simulink model "open_loop"  (R2021b)
settings: Solver=VariableStepAuto  StartTime=0.0  StopTime=2  RelTol=1e-3
undefined symbols (not defined in the file or in its folder): A, B, C, D
settings Model: Creator=Dawson  LastModifiedBy=Dawson

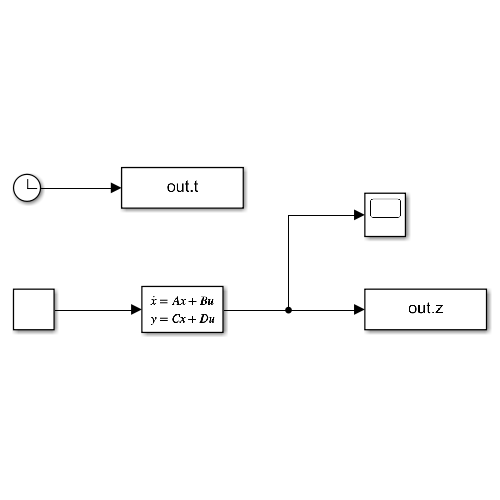
[thumbnail: Simulink's stored preview of the top-level diagram]
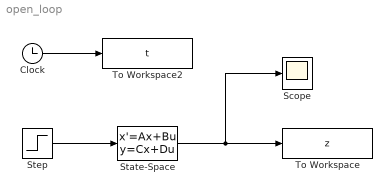
== system open_loop ==
  Clock : Clock
  Scope : Scope
  State-Space : StateSpace  A=A  B=B  C=C  D=D  InitialCondition=0
  Step : Step  Before=[0 0]  After=[10 0]  SampleTime=0
  To Workspace : ToWorkspace  VariableName=z  SaveFormat=Timeseries  SampleTime=-1
  To Workspace2 : ToWorkspace  VariableName=t  SampleTime=-1
      settings: Save2DSignal=2-D array (concatenate along first dimension)
  wires:
  Step/1 -> State-Space/1
  State-Space/1 -> To Workspace/1, Scope/1
  Clock/1 -> To Workspace2/1
